simulink model "BradleyWallHW2Unreal"  (R2024a)
settings: Solver=ode4  StartTime=0.0  StopTime=100  FixedStep=dt  MaxStep=0.01  RelTol=1e-12  AbsTol=1e-12  EnableMultiTasking=on
InitFcn:
  | clc
  | I = [3 0 0;0 4 0;0 0 2];
  | Iinv = I^-1;
  | dt = 0.005;
  | dtsim = 0.1;
  | wo = [0.001;0.001;1.001];
  | qo = [0;0;0;1];
  | Ho = [0;0;0];
StopFcn:
  | %close all
  | %omega = [(1/20)*cos(w.Time/200),-(1/20)*sin(w.Time/200),0.01*ones(length(w.Time),1)];
  | %plot(w.Time, omega-w.Data,'-')
  | %xlabel('Time, sec')
  | %ylabel('\omega_error, rad/s')
  | %legend('\omega_1','\omega_2','\omega_3','Location','northwest')
  | %Ho = I*wo;
  | %h = Ho/norm(Ho);
  | %wn = 1/200;
  | %wi = norm(Ho)/I(1,1);
  | %alpha = 0.5*wn*q.Time;
  | %beta = 0.5*wi*q.Time;
  | %qAct = [h(1)*cos(alpha).*sin(beta)+h(2)*sin(alpha).*sin(beta),...
  | %        h(2)*cos(alpha).*sin(beta)-h(1)*sin(alpha).*sin(beta),...
  | %        h(3)*cos(alpha).*sin(beta)+sin(alpha).*cos(beta),...
  | %        cos(alpha).*cos(beta)-h(3)*sin(alpha).*sin(beta)];
  | %figure
  | %plot(q.Time, qAct-q.Data,'-')
  | %xlabel('Time, sec')
  | %ylabel('q_{error}')
undefined symbols (not defined in the file): gray, Sim3dSensor
libraries: sim3dlib x4, vrlib x1, sharedutil x1
settings Model: Creator=wallb  LastModifiedBy=wallb
settings SolverCC: AutoScaleAbsTol=off  AlgebraicLoopSolver=TrustRegion
settings DataIOCC: LimitDataPoints=on  SaveFormat=Array  SignalLoggingSaveFormat=ModelDataLogs  ReturnWorkspaceOutputs=off
settings OptimizationCC: ExpressionDepthLimit=2147483647  LifeSpan=inf
settings DebuggingCC: UnderspecifiedInitializationDetection=Classic  MergeDetectMultiDrivingBlocksExec=none  SolverPrmCheckMsg=warning  FcnCallInpInsideContextMsg=warning  UnconnectedInputMsg=warning  UnconnectedOutputMsg=warning  UnconnectedLineMsg=warning  AllowSymbolicDim=off  StateNameClashWarn=warning  PregeneratedLibrarySubsystemCodeDiagnostic=none  SFUnexpectedBacktrackingDiag=warning  SFNoUnconditionalDefaultTransitionDiag=warning  SFExecutionAtInitializationDiag=none  ArithmeticOperatorsInVariantConditions=warning
settings HardwareCC: ProdBitPerPointer=32  ProdBitPerSizeT=32  ProdBitPerPtrDiffT=32  ProdLargestAtomicFloat=None  ProdIntDivRoundTo=Undefined  ProdEndianess=Unspecified  ProdWordSize=32  ProdHWDeviceType=32-bit Generic
settings ModelReferenceCC: EnableRefExpFcnMdlSchedulingChecks=on  PropagateSignalLabelsOutOfModel=off
settings SFSimCC: SimUseLocalCustomCode=off  CustomCodeUndefinedFunction=UseInterfaceOnly
settings RTWCC: RTWUseLocalCustomCode=off  GPUComputeCapability=3.5  DLArmComputeVersion=19.05
settings CodeAppCC: StateflowObjectComments=on
settings GRTTargetCC: TargetLangStandard=C89/C90 (ANSI)  CombineOutputUpdateFcns=off  GRTInterface=on
settings ConfigComp: CovMetricSettings=dw  CovSaveCumulativeToWorkspaceVar=on  CovSaveSingleToWorkspaceVar=on  CovExternalEMLEnable=off  CovSFcnEnable=off

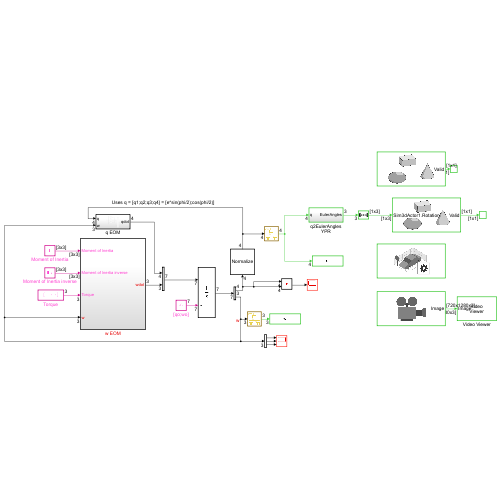
[thumbnail: Simulink's stored preview of the top-level diagram]
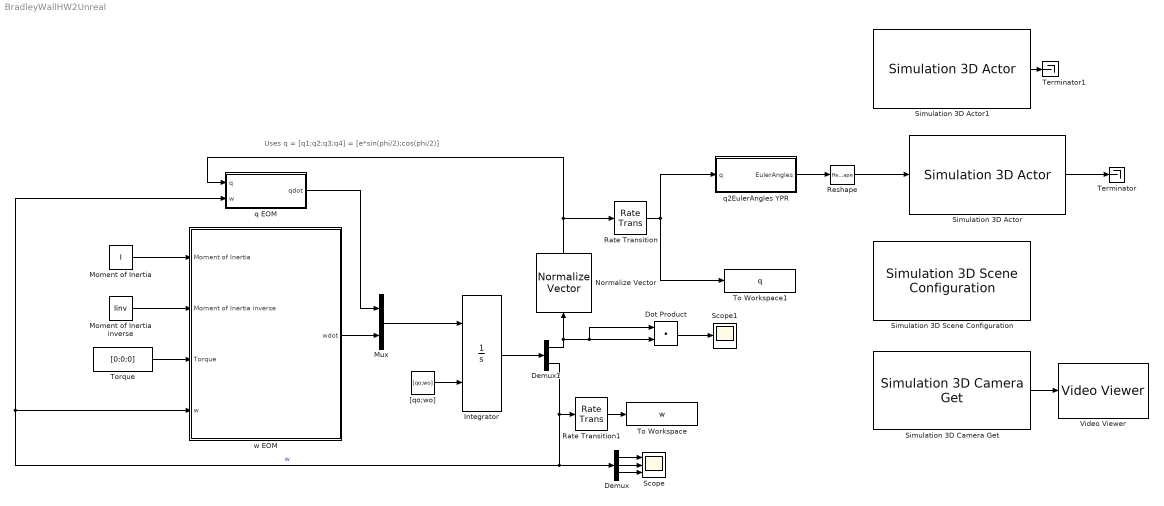
== system BradleyWallHW2Unreal ==
  note: Uses q = [q1;q2;q3;q4] = [e*sin(phi/2);cos(phi/2)]
  Demux : Demux  Outputs=3
  Demux1 : Demux  Outputs=2
  Dot Product : DotProduct  OutDataTypeStr=Inherit: Inherit via internal rule
  Integrator : Integrator  InitialConditionSource=external
  Moment of Inertia : Constant  Value=I
  Moment of Inertia inverse : Constant  Value=Iinv
  Mux : Mux  Inputs=2
  Normalize Vector : vrlib/Utilities/Normalize Vector  maxzero=0
  Rate Transition : RateTransition  InitialCondition=qo  OutPortSampleTime=dtsim
  Rate Transition1 : RateTransition  InitialCondition=wo  OutPortSampleTime=dtsim
  Reshape : Reshape  OutputDimensionality=Row vector (2-D)
  Scope : Scope  NumInputPorts=3
  Scope1 : Scope
  Simulation 3D Actor : sim3dlib/Simulation 3D Actor  Priority=1  ActorName=Sim3dActor1  ParentName=Scene Origin  Operation=Create at setup  InitScriptText=|  SampleTime=-1  Translation=[0 0 0]  Rotation=[0 0 0]  Scale=[1 1 1]  InputsText=Sim3dActor1.Rotation  aMode=5  ActorTag=Sim3dActor1  ActorType=Sim3dActor  ID=1
      | % Reserved keywords:
      | % - Actor : handle to this actor object
      | % - World : handle to the world object
      | 
      | % Examples:
      | 
      | % Create a primitive geometry (optional)
      | % createShape(Actor, 'box', [1 1 1]);
      | 
      | % Initialize values (optional)
      | % Actor.Physics = true;
      | % Actor.Color = [1 0 0];
  Simulation 3D Actor1 : sim3dlib/Simulation 3D Actor  Priority=1  ActorName=Sim3dActor2  ParentName=Scene Origin  Operation=Create at setup  InitScriptText=|  SampleTime=-1  Translation=[0 0 0]  Rotation=[0 0 0]  Scale=[1 1 1]  aMode=5  ActorTag=Sim3dActor2  ActorType=Sim3dActor  ID=2
      | pointLight1 = sim3d.Light(ActorName='PointLight1',LightType='PointLight');
      | pointLight1.Intensity = 5000000;
      | pointLight1.AttenuationRadius = 2000;
      | pointLight1.Translation = [0 0 100];
      | pointLight1.LightColor = [1 1 1];
      | 
      | pointLight2 = sim3d.Light(ActorName='PointLight2',LightType='PointLight');
      | pointLight2.Intensity = 5000000;
      | pointLight2.AttenuationRadius = 2000;
      | pointLight2.Translation = [0 0 -100];
      | pointLight2.LightColor = [1 1 1];
      | 
      | pointLight3 = sim3d.Light(ActorName='PointLight3',LightType='PointLight');
      | pointLight3.Intensity = 5000000;
      | pointLight3.AttenuationRadius = 2000;
      | pointLight3.Translation = [0 100 0];
      | pointLight3.LightColor = [1 1 1];
      | 
      | pointLight4 = sim3d.Light(ActorName='PointLight4',LightType='PointLight');
      | pointLight4.Intensity = 5000000;
      | pointLight4.AttenuationRadius = 2000;
      | pointLight4.Translation = [0 -100 0];
      | pointLight4.LightColor = [1 1 1];
      | 
      | pointLight5 = sim3d.Light(ActorName='PointLight5',LightType='PointLight');
      | pointLight5.Intensity = 5000000;
      | pointLight5.AttenuationRadius = 2000;
      | pointLight5.Translation = [100 0 0];
      | pointLight5.LightColor = [1 1 1];
      | 
      | pointLight6 = sim3d.Light(ActorName='PointLight6',LightType='PointLight');
      | pointLight6.Intensity = 5000000;
      | pointLight6.AttenuationRadius = 2000;
      | pointLight6.Translation = [-100 0 0];
      | pointLight6.LightColor = [1 1 1];
      | 
      | add(World,pointLight1,Actor);
      | add(World,pointLight2,Actor);
      | add(World,pointLight3,Actor);
      | add(World,pointLight4,Actor);
      | add(World,pointLight5,Actor);
      | add(World,pointLight6,Actor);
  Simulation 3D Camera Get : sim3dlib/Simulation 3D Camera Get  Priority=1  sensorTag=Sim3dSensor�  sensorId=3  sensorName=Sim3dSensor�  vehTagList={'Scene Origin';'Sim3dActor1';'Sim3dActor2'}  vehTag=Scene Origin  mountLoc=Origin  offsetFlag=on  tmountOffset=[0, 0, -300]  rmountOffset=[90, -90, 0]  HorizontalResolution=1280  VerticalResolution=720  HorizontalFOV=60  SampleTime=-1  mountPoint=[0 0 -300]  mountOrientation=[90 90 0]  aMode=5  ID=3
      settings: LibrarySourceBlock=sl3dlib/Simulation 3D/Utilities/Simulation 3D Camera Get
  Simulation 3D Scene Configuration : sim3dlib/Simulation 3D Scene Configuration  Priority=0  ProjectFormat=Default Scenes  SceneDesc=Empty scene  ProjectName=C:\Program Files\MATLAB\R2024a\toolbox\shared\sim3d_projects\automotive_project_windows\UE\WindowsNoEditor\VehicleSimulation.exe  ScenePath=/Game/Maps/HwStrght  UEProjPath=C:\Users\brady\Documents\Unreal Projects\MyProject\MyProject.uproject  EnableOpenDRIVE=off  vehTagList={'Custom';'Scene Origin';'Sim3dActor1';'Sim3dActor2'}  vehTag=Custom  FreeCameraInitialTranslation=[0, 0, -300]  FreeCameraDefaultInitialTranslation=[-6, 0, 2]  FreeCameraInitialRotation=[90, -90, 0]  FreeCameraDefaultInitialRotation=[0, -15, 0]  OpVisEn=off  Ts=dtsim  EnableWindow=off  EnableRemoteAccess=off  EnableWeather=on  SunAzimuth=90  SunAltitude=-90.0  EnableGeospatialSun=off  Latitude=0  Longitude=0  Date=2023-01-01  Time=10:30:00  GeoTimeZone=-5.0  SunDaylightSaving=off  wind=1  clouds=10.0  EnableVolumetricClouds=off  CloudCoverage=0  CloudAltitude=6  fog=0  rain=0  RaindropsEffect=off  SnowDensity=0  EnableGeospatial=off  UseTrueOrigin=off  OriginHeight=200  OriginLatitude=40.744652  OriginLongitude=-73.988864  MapStyle=Aerial  AdditionalAssetIDs=[]  UseAdvancedSunSky=off  SolarTime=11  TimeZone=-5  Day=21  Month=9  Year=2022  UseDaylightSavingTime=on  DSTStartDay=10  DSTStartMonth=3  DSTEndDay=3  DSTEndMonth=11  DSTSwitchHour=2  sensorTag=MainCamera1  sensorId=1  sensorName=MainCamera1  mountLoc=Origin  offsetFlag=off  tmountOffset=[0, 0, 0]  rmountOffset=[0, 0, 0]  HorizontalResolution=1280  VerticalResolution=720  HorizontalFOV=60  mountPoint=[0 0 0]  mountOrientation=[0 0 0]  aMode=5  ID=1  GeoTrigger=Inactive
      settings: LibrarySourceBlock=sl3dlib/Simulation 3D/Environment/Simulation 3D Scene Configuration
  Terminator : Terminator
  Terminator1 : Terminator
  To Workspace : ToWorkspace  VariableName=w  SaveFormat=Timeseries  SampleTime=-1
  To Workspace1 : ToWorkspace  VariableName=q  SaveFormat=Timeseries  SampleTime=-1
  Torque : Constant  Value=[0;0;0]
  Video Viewer : VideoViewer  colormapValue=gray(256)  FigPos=[630 867 827 583]
  "[qo;wo]" : Constant  Value=[qo;wo]
  q EOM : Subsystem
  q2EulerAngles YPR : Subsystem
  w EOM : Subsystem
  wires:
  Moment of Inertia/1 -> w EOM/1(Moment of Inertia)
  Moment of Inertia inverse/1 -> w EOM/2(Moment of Inertia inverse)
  Torque/1 -> w EOM/3(Torque)
  "[qo;wo]"/1 -> Integrator/2
  Demux1/1 -> Dot Product/2, Dot Product/1, Normalize Vector/1
  Demux/1 -> Scope/1
  Demux/2 -> Scope/2
  Demux/3 -> Scope/3
  Dot Product/1 -> Scope1/1
  w EOM/1(wdot) -> Mux/2
  Mux/1 -> Integrator/1
  Integrator/1 -> Demux1/1
  Demux1/2 -> Demux/1, q EOM/2(w), w EOM/4(w), Rate Transition1/1  "w"
  q EOM/1(qdot) -> Mux/1
  Normalize Vector/1 -> Rate Transition/1, q EOM/1(q)
  Rate Transition1/1 -> To Workspace/1
  q2EulerAngles YPR/1(EulerAngles) -> Reshape/1
  Simulation 3D Actor/1 -> Terminator/1
  Simulation 3D Actor1/1 -> Terminator1/1
  Simulation 3D Camera Get/1 -> Video Viewer/1
  Rate Transition/1 -> q2EulerAngles YPR/1(q), To Workspace1/1
  Reshape/1 -> Simulation 3D Actor/1

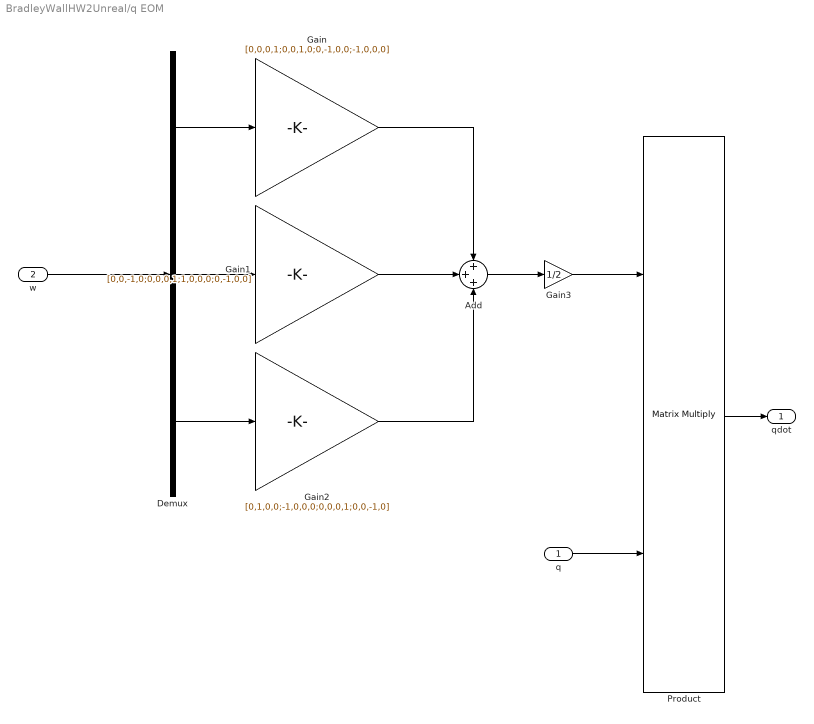
== system BradleyWallHW2Unreal/q EOM ==
  q : Inport
  w : Inport  Port=2
  Add : Sum  Inputs=+++
  Demux : Demux  Outputs=3
  Gain : Gain  Gain=[0,0,0,1;0,0,1,0;0,-1,0,0;-1,0,0,0]
  Gain1 : Gain  Gain=[0,0,-1,0;0,0,0,1;1,0,0,0;0,-1,0,0]
  Gain2 : Gain  Gain=[0,1,0,0;-1,0,0,0;0,0,0,1;0,0,-1,0]
  Gain3 : Gain  Gain=1/2
  Product : Product  Multiplication=Matrix(*)
  qdot : Outport
  wires:
  w/1 -> Demux/1
  Demux/1 -> Gain/1
  Demux/2 -> Gain1/1
  Demux/3 -> Gain2/1
  Gain1/1 -> Add/2
  Gain/1 -> Add/1
  Gain2/1 -> Add/3
  q/1 -> Product/2
  Product/1 -> qdot/1
  Add/1 -> Gain3/1
  Gain3/1 -> Product/1

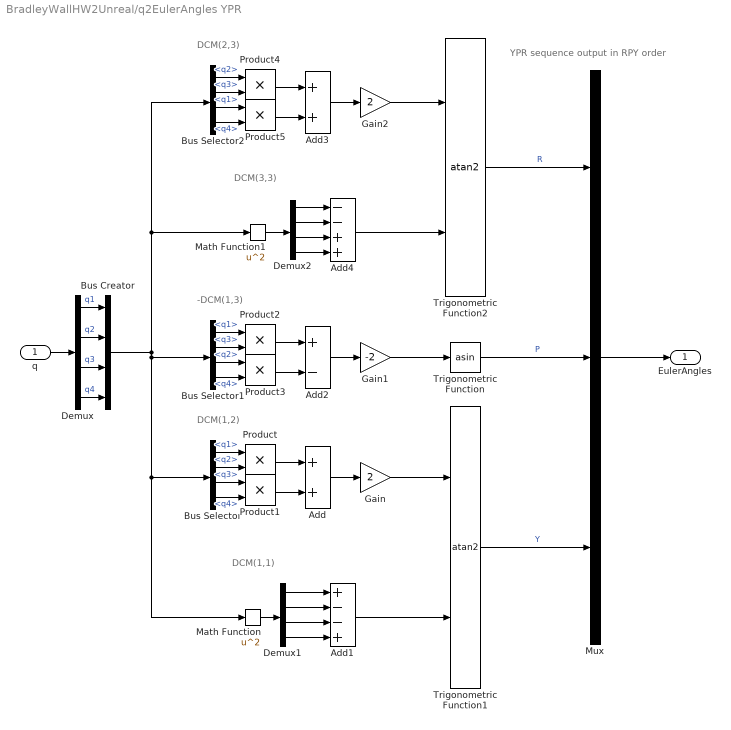
== system BradleyWallHW2Unreal/q2EulerAngles YPR ==
  note: YPR sequence output in RPY order
  note: DCM(3,3)
  note: DCM(2,3)
  note: -DCM(1,3)
  note: DCM(1,1)
  note: DCM(1,2)
  q : Inport
  Add : Sum
  Add1 : Sum  Inputs=+--+
  Add2 : Sum  Inputs=+-
  Add3 : Sum
  Add4 : Sum  Inputs=--++
  Bus Creator : BusCreator  Inputs=4
  Bus Selector : BusSelector  OutputSignals=q1,q2,q3,q4
  Bus Selector1 : BusSelector  OutputSignals=q1,q3,q2,q4
  Bus Selector2 : BusSelector  OutputSignals=q2,q3,q1,q4
  Demux : Demux
  Demux1 : Demux
  Demux2 : Demux
  Gain : Gain  Gain=2
  Gain1 : Gain  Gain=-2
  Gain2 : Gain  Gain=2
  Math Function : Math  Operator=square
  Math Function1 : Math  Operator=square
  Mux : Mux  Inputs=3
  Product{,1..5} (6 alike) : Product
  Trigonometric Function : Trigonometry  Operator=asin
  Trigonometric Function1 : Trigonometry  Operator=atan2
  Trigonometric Function2 : Trigonometry  Operator=atan2
  EulerAngles : Outport  VectorParamsAs1DForOutWhenUnconnected=off
  wires:
  Add4/1 -> Trigonometric Function2/2
  Add1/1 -> Trigonometric Function1/2
  Gain/1 -> Trigonometric Function1/1
  Gain2/1 -> Trigonometric Function2/1
  Trigonometric Function2/1 -> Mux/1  "R"
  Trigonometric Function/1 -> Mux/2  "P"
  Trigonometric Function1/1 -> Mux/3  "Y"
  q/1 -> Demux/1
  Demux/1 -> Bus Creator/1  "q1"
  Demux/2 -> Bus Creator/2  "q2"
  Demux/3 -> Bus Creator/3  "q3"
  Demux/4 -> Bus Creator/4  "q4"
  Gain1/1 -> Trigonometric Function/1
  Bus Selector/3 -> Product1/1  "<q3>"
  Bus Selector/2 -> Product/2  "<q2>"
  Product1/1 -> Add/2
  Add/1 -> Gain/1
  Bus Selector/1 -> Product/1  "<q1>"
  Bus Selector/4 -> Product1/2  "<q4>"
  Product/1 -> Add/1
  Demux1/1 -> Add1/1
  Demux1/4 -> Add1/4
  Demux1/2 -> Add1/2
  Demux1/3 -> Add1/3
  Math Function/1 -> Demux1/1
  Bus Selector1/3 -> Product3/1  "<q2>"
  Product2/1 -> Add2/1
  Bus Selector1/4 -> Product3/2  "<q4>"
  Bus Selector1/1 -> Product2/1  "<q1>"
  Bus Selector1/2 -> Product2/2  "<q3>"
  Add2/1 -> Gain1/1
  Product3/1 -> Add2/2
  Bus Selector2/4 -> Product5/2  "<q4>"
  Bus Selector2/3 -> Product5/1  "<q1>"
  Bus Selector2/2 -> Product4/2  "<q3>"
  Bus Selector2/1 -> Product4/1  "<q2>"
  Product4/1 -> Add3/1
  Add3/1 -> Gain2/1
  Product5/1 -> Add3/2
  Demux2/1 -> Add4/1
  Demux2/4 -> Add4/4
  Demux2/2 -> Add4/2
  Demux2/3 -> Add4/3
  Math Function1/1 -> Demux2/1
  Bus Creator/1 -> Math Function/1, Bus Selector/1, Bus Selector1/1, Bus Selector2/1, Math Function1/1
  Mux/1 -> EulerAngles/1

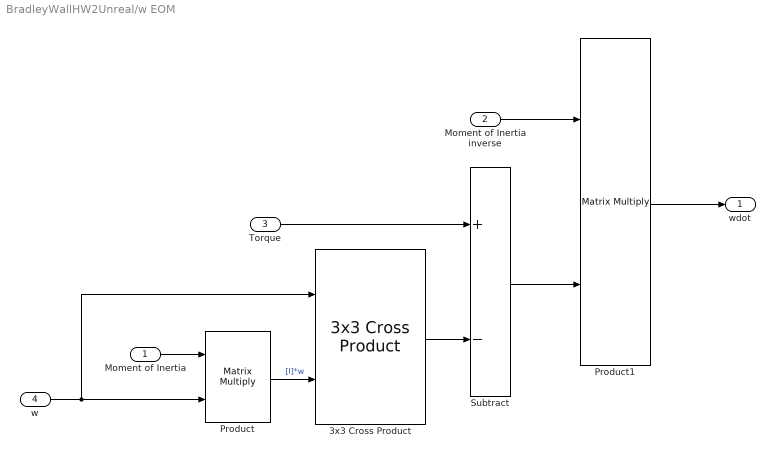
== system BradleyWallHW2Unreal/w EOM ==
  Moment of Inertia : Inport
  Moment of Inertia inverse : Inport  Port=2
  Torque : Inport  Port=3
  w : Inport  Port=4
  3x3 Cross Product : sharedutil/3x3 Cross Product  aMode=aMode
  Product : Product  Multiplication=Matrix(*)  RndMeth=Zero
  Product1 : Product  Multiplication=Matrix(*)  RndMeth=Zero
  Subtract : Sum  Inputs=+-
  wdot : Outport  VectorParamsAs1DForOutWhenUnconnected=off
  wires:
  Moment of Inertia/1 -> Product/1
  Torque/1 -> Subtract/1
  3x3 Cross Product/1 -> Subtract/2
  Moment of Inertia inverse/1 -> Product1/1
  Subtract/1 -> Product1/2
  Product1/1 -> wdot/1
  Product/1 -> 3x3 Cross Product/2  "[I]*w"
  w/1 -> 3x3 Cross Product/1, Product/2
